simulink model "projectCE1"  (R2024a)
settings: Solver=VariableStepAuto  StartTime=0.0  StopTime=0.1  FixedStep=1/Fs  RelTol=1e-9
model workspace (MATLAB code in the model file):
  | [audioData, sampleRate] = audioread('filename.wav');
values from neighbouring files (symbols this model uses):
  f1_AM = 140000    [proyecto.m]
  f2_AM = 180000    [proyecto.m]
  f3_AM = 220000    [proyecto.m]
  fc_FM = 1e6    (= 1000000)    [proyecto.m]
  Fs1 = 500e3    (= 500000)    [proyecto.m]
  Kf = 72e3    (= 72000)    [proyecto.m]
libraries: dspfdesign x3
settings Model: Creator=nagel  LastModifiedBy=nagel

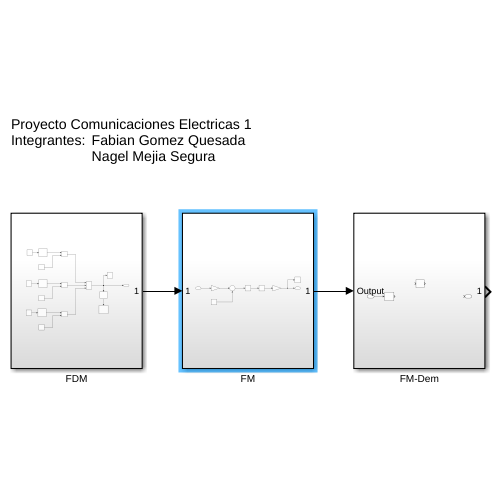
[thumbnail: Simulink's stored preview of the top-level diagram]
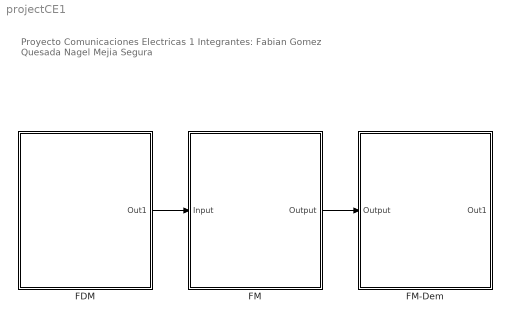
== system projectCE1 ==
  note: Proyecto Comunicaciones Electricas 1
      | Integrantes: Fabian Gomez Quesada
      | Nagel Mejia Segura
  FDM : Subsystem
  FM : Subsystem
  FM-Dem : Subsystem
  wires:
  FDM/1(Out1) -> FM/1(Input)
  FM/1(Output) -> FM-Dem/1(Output)

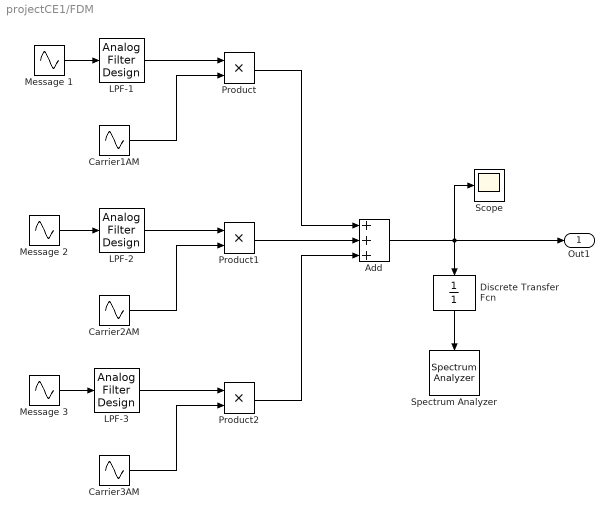
== system projectCE1/FDM ==
  Add : Sum  Inputs=+++
  Carrier1AM : Sin  Frequency=2*pi*f1_AM  SampleTime=1/Fs1
  Carrier2AM : Sin  Frequency=2*pi*f2_AM  SampleTime=1/Fs1
  Carrier3AM : Sin  Frequency=2*pi*f3_AM  SampleTime=1/Fs1
  Discrete Transfer Fcn : DiscreteTransferFcn  Denominator=[1]
  LPF-1 : dspfdesign/Analog Filter Design  method=Butterworth  filttype=Lowpass  N=8  Wlo=2*pi*15000  Whi=80  Rp=2  Rs=40
  LPF-2 : dspfdesign/Analog Filter Design  method=Butterworth  filttype=Lowpass  N=8  Wlo=2*pi*15000  Whi=80  Rp=2  Rs=40
  LPF-3 : dspfdesign/Analog Filter Design  method=Butterworth  filttype=Lowpass  N=8  Wlo=2*pi*15000  Whi=80  Rp=2  Rs=40
  Message 1 : Sin  Amplitude=2  Frequency=2*pi*780  SampleTime=1/Fs1
  Message 2 : Sin  Frequency=2*pi*5000  SampleTime=1/Fs1
  Message 3 : Sin  Amplitude=2  Frequency=2*pi*2000  SampleTime=1/Fs1
  Product : Product
  Product1 : Product
  Product2 : Product
  Scope : Scope
  Spectrum Analyzer : SpectrumAnalyzer  WindowPosition=[524.000000,200.000000,857.000000,500.000000,]  Visible=on  ScopeFrameLocation=window  SampleRate=500000  PlotAsTwoSidedSpectrum=off  RBWSource=Property  RBW=50  NumTapsPerBand=78  FilterSharpness=1  Span=250000  CenterFrequency=125000  StartFrequency=0  StopFrequency=250000  YLimits=[-58.14382164,36.44810028]  SelectedToolstripTab=spectrumAnalyzerToolstrip.estimationTab
  Out1 : Outport
  wires:
  Message 3/1 -> LPF-3/1
  Product2/1 -> Add/3
  Carrier1AM/1 -> Product/2
  Carrier2AM/1 -> Product1/2
  Carrier3AM/1 -> Product2/2
  Product1/1 -> Add/2
  Product/1 -> Add/1
  Message 1/1 -> LPF-1/1
  LPF-1/1 -> Product/1
  LPF-2/1 -> Product1/1
  LPF-3/1 -> Product2/1
  Message 2/1 -> LPF-2/1
  Add/1 -> Out1/1, Discrete Transfer Fcn/1, Scope/1
  Discrete Transfer Fcn/1 -> Spectrum Analyzer/1

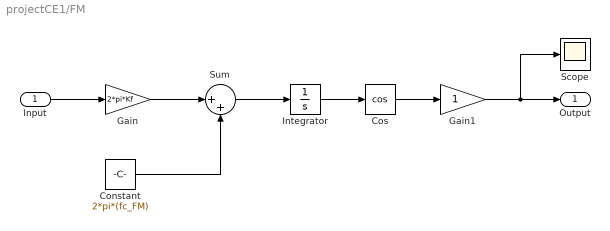
== system projectCE1/FM ==
  Input : Inport
  Constant : Constant  Value=2*pi*(fc_FM)
  Cos : Trigonometry  Operator=cos
  Gain : Gain  Gain=2*pi*Kf
  Gain1 : Gain
  Integrator : Integrator
  Scope : Scope
  Sum : Sum  Inputs=|++
  Output : Outport
  wires:
  Gain/1 -> Sum/1
  Constant/1 -> Sum/2
  Sum/1 -> Integrator/1
  Integrator/1 -> Cos/1
  Cos/1 -> Gain1/1
  Input/1 -> Gain/1
  Gain1/1 -> Output/1, Scope/1

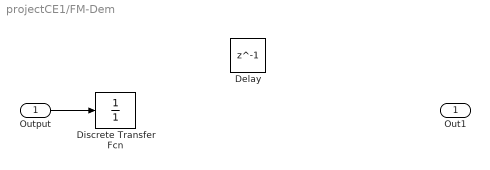
== system projectCE1/FM-Dem ==
  Output : Inport
  Delay : Delay  DelayLength=1  InitialCondition=0
  Discrete Transfer Fcn : DiscreteTransferFcn  Denominator=[1]
  Out1 : Outport
  wires:
  Output/1 -> Discrete Transfer Fcn/1
